simulink model "PS3"  (R2024a)
settings: Solver=VariableStepAuto  StartTime=0.0  StopTime=10.0  RelTol=1e-3
settings Model: Creator=LAPTOP  LastModifiedBy=LAPTOP

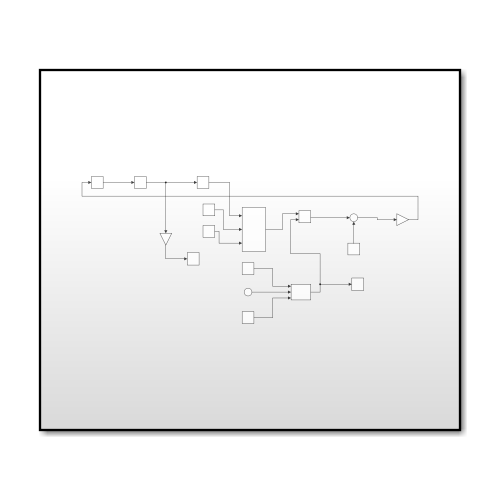
[thumbnail: Simulink's stored preview of the top-level diagram]
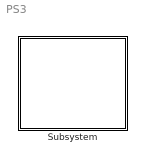
== system PS3 ==
  Subsystem : Subsystem

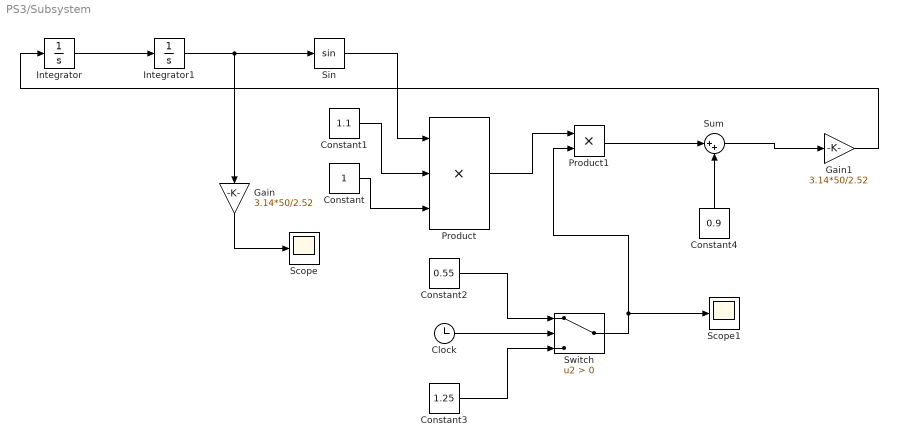
== system PS3/Subsystem ==
  Clock : Clock
  Constant : Constant
  Constant1 : Constant  Value=1.1
  Constant2 : Constant  Value=0.55
  Constant3 : Constant  Value=1.25
  Constant4 : Constant  Value=0.9
  Gain : Gain  Gain=3.14*50/2.52
  Gain1 : Gain  Gain=3.14*50/2.52
  Integrator : Integrator
  Integrator1 : Integrator
  Product : Product  Inputs=3
  Product1 : Product
  Scope : Scope
  Scope1 : Scope
  Sin : Trigonometry
  Sum : Sum  Inputs=|++
  Switch : Switch  Criteria=u2 > Threshold  SaturateOnIntegerOverflow=off  InputSameDT=off
  wires:
  Integrator/1 -> Integrator1/1
  Integrator1/1 -> Gain/1, Sin/1
  Gain/1 -> Scope/1
  Sin/1 -> Product/1
  Constant1/1 -> Product/2
  Constant/1 -> Product/3
  Constant2/1 -> Switch/1
  Clock/1 -> Switch/2
  Constant3/1 -> Switch/3
  Product/1 -> Product1/1
  Switch/1 -> Product1/2, Scope1/1
  Product1/1 -> Sum/1
  Constant4/1 -> Sum/2
  Sum/1 -> Gain1/1
  Gain1/1 -> Integrator/1
